simulink model "Y6MultirotorOpenLoopModelSimulation2"  (R2019b)
settings: Solver=VariableStepAuto  StartTime=0.0  StopTime=60  RelTol=1e-3
values from neighbouring files (symbols this model uses):
  U_e = sqrt(((M*g)/(3*(Kthrust+(Kw*Kthrust)))))    [ControlDesign14States.m]    (also in ControlDesign18States.m = ((-6*Kthrust2) + sqrt((6*Kthrust2)^2 - (4*(-M*g)*(3*Kw*Kthru; ControlDesign8States.m = ((-6*Kthrust2) + sqrt((6*Kthrust2)^2 - (4*(-M*g)*(3*Kw*Kthru; Dynamics.m = ((-6*Kthrust2) + sqrt((6*Kthrust2)^2 - (4*(-M*g)*(3*Kw*Kthru; Equations_Of_Motion.m = 1500)
settings Model: Creator=oscar  LastModifiedBy=alexd
settings SolverCC: AlgebraicLoopSolver=LineSearch
settings DataIOCC: ReturnWorkspaceOutputs=off
settings DebuggingCC: ArithmeticOperatorsInVariantConditions=warning
settings SFSimCC: SimUseLocalCustomCode=off  CustomCodeUndefinedFunction=UseInterfaceOnly
settings RTWCC: RTWUseLocalCustomCode=off

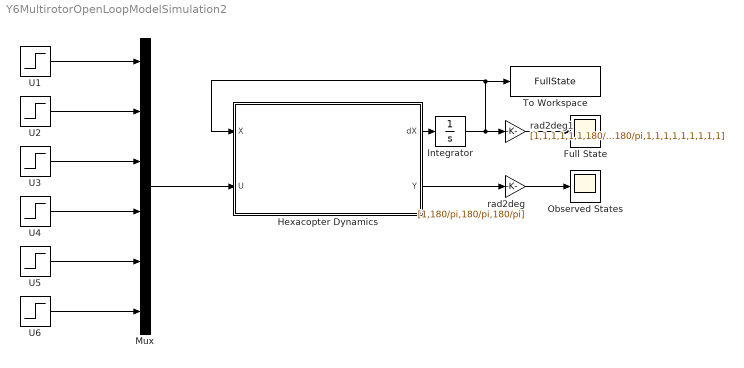
== system Y6MultirotorOpenLoopModelSimulation2 ==
  Full State : Scope
  Hexacopter Dynamics : MATLAB Function  TreatAsAtomicUnit=on
  Integrator : Integrator  InitialCondition=[0;0;0;0;0;0;0;0;0;0;0;0;0;0;0;0;0;0]
  Mux : Mux  Inputs=6
  Observed States : Scope
  To Workspace : ToWorkspace  VariableName=FullState  SaveFormat=Timeseries  SampleTime=-1
  U{1..6} (6 alike) : Step  Time=0  After=U_e  SampleTime=0
  rad2deg : Gain  Gain=[1,180/pi,180/pi,180/pi]  SaturateOnIntegerOverflow=on  OutDataTypeStr=Inherit: Same as input  ParamDataTypeStr=Inherit: Same as input
  rad2deg1 : Gain  Gain=[1,1,1,1,1,1,180/pi,180/pi,180/pi,1,1,1,1,1,1,1,1,1]  SaturateOnIntegerOverflow=on  OutDataTypeStr=Inherit: Same as input  ParamDataTypeStr=Inherit: Same as input
  wires:
  Hexacopter Dynamics/1(dX) -> Integrator/1
  Integrator/1 -> To Workspace/1, Hexacopter Dynamics/1(X), rad2deg1/1
  U1/1 -> Mux/1
  Hexacopter Dynamics/2(Y) -> rad2deg/1
  U2/1 -> Mux/2
  U4/1 -> Mux/4
  U3/1 -> Mux/3
  rad2deg/1 -> Observed States/1
  rad2deg1/1 -> Full State/1
  Mux/1 -> Hexacopter Dynamics/2(U)
  U5/1 -> Mux/5
  U6/1 -> Mux/6

== matlab function Y6MultirotorOpenLoopModelSimulation2/Hexacopter Dynamics ==
  data: dX output; X input; U input; Y output
function [dX,Y]  = Hexacopter_Dynamics(X,U)
%% Mass of the Multirotor in Kilograms as taken from the CAD

M = 2100/1000; 
g = 9.81;

%% Dimensions of Multirotor

L1 = 22/100; % along X-axis Distance from left and right motor pair to center of mass
L2 = 15/100; % along Y-axis Vertical Distance from left and right motor pair to center of mass
L3 = 30/100; % along Y-axis Distance from motor pair to center of mass

%%  Mass Moment of Inertia as Taken from the CAD

Ixx = 3.094E+05;
Ixy = 45.147;
Ixz = 2.309;
Iyx = 45.147;
Iyy = 4.204E+05;
Iyz = 832.833;
Izx = 2.309;
Izy = 832.833;
Izz = 1.464E+05;

%% Inertia Matrix and Diagolalisation CAD model coordinate system rotated 90 degrees about X

I = [Izx Izy Izz;
     Ixx Ixy Ixz;
     Iyx Iyy Iyz];
 
Idiag = diag(I)/10000;
 
Ixx = Idiag(1);
Iyy = Idiag(2);
Izz = Idiag(3);

%% Motor Thrust and Torque Constants (To be determined experimentally)

Kw = 0.85;
Ktau =  3.46*(10^-8);
Kthrust =  1.0155*(10^-7) ;
Kthrust2 = -1.0327*(10^-4);
Mtau = 0.038; %0.09;
Ku = 82.3;%0.0667;%0.014;

%% Air resistance damping coeeficients

Dxx = 0.02;
Dyy = 0.02;
Dzz = 0.1;

%% X = [x xdot y ydot z zdot phi phidot theta thetadot psi psidot w1 w2 w3 w4 w5 w6]

x = X(1);
xdot = X(2);
y = X(3);
ydot = X(4);
z = X(5);
zdot = X(6);

phi = X(7); 
theta = X(8);
psi = X(9);

p = X(10);
q = X(11);
r = X(12);

w1 = X(13);
w2 = X(14);
w3 = X(15);
w4 = X(16);
w5 = X(17);
w6 = X(18);

%% Initialise Outputs

dX = zeros(18,1);
Y = zeros(4,1);

%% Motor Dynamics: dX = [w1dot w2dot w3dot w4dot w5dot w6dot], U = Duty Cycle of the pwm signal 0-100%

dX(13) = -(1/Mtau)*w1 + (Ku/Mtau)*U(1);
dX(14) = -(1/Mtau)*w2 + (Ku/Mtau)*U(2);
dX(15) = -(1/Mtau)*w3 + (Ku/Mtau)*U(3);
dX(16) = -(1/Mtau)*w4 + (Ku/Mtau)*U(4);
dX(17) = -(1/Mtau)*w5 + (Ku/Mtau)*U(5);
dX(18) = -(1/Mtau)*w6 + (Ku/Mtau)*U(6);

%% Motor Forces and Torques

F = zeros(6,1);
T = zeros(6,1);

F(1)= Kw*Kthrust*(w1^2) + Kthrust2*w1;
F(2)= Kthrust*(w2^2) + Kthrust2*w2;
F(3)= Kw*Kthrust*(w3^2)+ Kthrust2*w3;
F(4)= Kthrust*(w4^2) + Kthrust2*w4;
F(5)= Kw*Kthrust*(w5^2) + Kthrust2*w5;
F(6)= Kthrust*(w6^2) + Kthrust2*w6;

T(1)= Ktau*(w1^2);
T(2)= -Ktau*(w2^2);
T(3)= -Ktau*(w3^2);
T(4)= Ktau*(w4^2);
T(5)= Ktau*(w5^2);
T(6)= -Ktau*(w6^2);

Fn = sum(F);
Tn = sum(T);

%% First Order Direvatives dX = [xdot ydot zdot phidot thetadot psidot]

dX(1) = X(2);
dX(3) = X(4);
dX(5) = X(6);
dX(7) = p + q*(sin(phi)*tan(theta)) + r*(cos(phi)*tan(theta));
dX(8) = q*cos(phi) - r*sin(phi);
dX(9) = q*(sin(phi)/cos(theta)) + r*(cos(phi)/cos(theta));

%% Second Order Direvatives: dX = [xddot yddot zddot pdot qdot rdot]

dX(2) = Fn/M*(cos(phi)*sin(theta)*cos(psi)) + Fn/M*(sin(phi)*sin(psi)) - (Dxx/M)*xdot;
dX(4) = Fn/M*(cos(phi)*sin(theta)*sin(psi)) - Fn/M*(sin(phi)*cos(psi)) - (Dyy/M)*ydot;
dX(6) = Fn/M*(cos(phi)*cos(theta)) - g - (Dzz/M)*zdot;

dX(10) = (L1/Ixx)*((F(1)+F(2)) - (F(3)+F(4))) - ((Izz-Iyy)/Ixx)*(r*q); 
dX(11) = (L3/Iyy)*(F(5)+F(6)) - (L2/Iyy)*(F(1)+F(2)+F(3)+F(4)) - ((Izz-Ixx)/Iyy)*(p*r);
dX(12) = Tn/Izz - ((Iyy-Ixx)/Izz)*(p*q);

%% Measured States

Y(1) = z;
Y(2) = phi;
Y(3) = theta;
Y(4) = psi;

end
